simulink model "tst_bus_name_with_comma"  (Simulink 8.0)
settings: Solver=ode45  StartTime=0.0  StopTime=10.0  RelTol=1e-3
settings Model: Creator=Marci  LastModifiedBy=transima

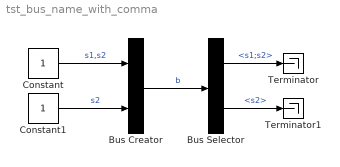
== system tst_bus_name_with_comma ==
  Bus Creator : BusCreator  Inputs=2
  Bus Selector : BusSelector  OutputSignals=s1;s2,s2
  Constant : Constant
  Constant1 : Constant
  Terminator : Terminator
  Terminator1 : Terminator
  wires:
  Constant1/1 -> Bus Creator/2  "s2"
  Constant/1 -> Bus Creator/1  "s1,s2"
  Bus Creator/1 -> Bus Selector/1  "b"
  Bus Selector/1 -> Terminator/1  "<s1;s2>"
  Bus Selector/2 -> Terminator1/1  "<s2>"
